simulink model "matlab_ppg_v2"  (R2018a)
settings: Solver=FixedStepAuto  StartTime=0.0  StopTime=inf  RelTol=1e-3  EnableMultiTasking=on
libraries: dspstat3 x5, arduinolib x1, dspsrcs4 x1
settings Model: ExtModeTrigDuration=2  Creator=Na-Teng  LastModifiedBy=Na-Teng
settings OptimizationCC: EnhancedBackFolding=on  PassReuseOutputArgsAs=Individual arguments  MaxStackSize=64  OptimizeBlockOrder=speed  DifferentSizesBufferReuse=on  OptimizationCustomize=off
settings DebuggingCC: ParameterTunabilityLossMsg=error
settings HardwareCC: ProdBitPerInt=16  ProdBitPerPointer=16  ProdBitPerSizeT=16  ProdBitPerPtrDiffT=16  ProdLargestAtomicFloat=None  ProdWordSize=8  ProdHWDeviceType=Atmel->AVR
settings SFSimCC: MATLABDynamicMemAlloc=off
settings RTWCC: SystemTargetFile=ert.tlc  HardwareBoard=Arduino Mega 2560  TLCOptions=-aInlineSetEventsForThisBaseRateFcn=TLC_FALSE -aSuppressMultiTaskScheduler=TLC_FALSE -aRateBasedStepFcn=1  TemplateMakefile=ert_default_tmf  GenerateReport=on  Toolchain=Arduino AVR  BuildConfiguration=Faster Runs  IncludeHyperlinkInReport=on  LaunchReport=on  GenerateTraceInfo=on  GenerateTraceReport=on  GenerateTraceReportSl=on  GenerateTraceReportSf=on  GenerateTraceReportEml=on
settings CodeAppCC: ForceParamTrailComments=on  IgnoreCustomStorageClasses=off  OperatorAnnotations=on  SimulinkDataObjDesc=on  SFDataObjDesc=on  InsertBlockDesc=on
settings ERTTargetCC: SupportContinuousTime=on  SupportVariableSizeSignals=on

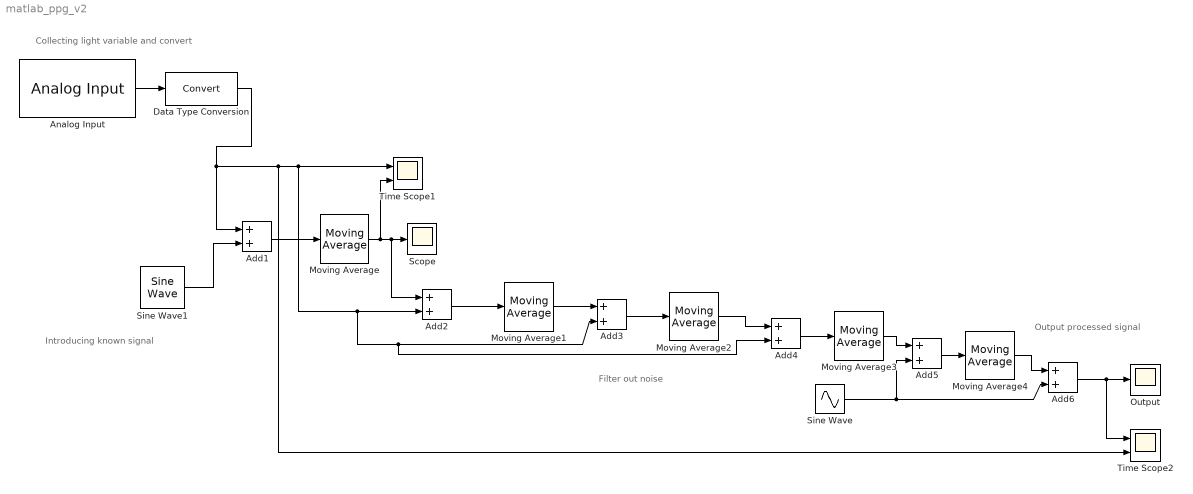
== system matlab_ppg_v2 ==
  note: Output processed signal
  note: Filter out noise
  note: Introducing known signal
  note: Collecting light variable and convert
  Add{1..6} (6 alike) : Sum
  Analog Input : arduinolib/Analog Input  pinNumber=4  ReadResultsOnly=off  ConversionTriggerSource=Software  ExternalTriggerType=uint32(0)  OutputDataType=uint16  EnableConversionCompleteNotify=off  EnableOuputStatus=off  SampleTime=0.001  blockPlatform=arduino
  Data Type Conversion : DataTypeConversion
  Moving Average{,1..4} (5 alike) : dspstat3/Moving Average  Method=Exponential weighting  ForgettingFactorPort=off  SpecifyWindowLength=on  WindowLength=12  ForgettingFactor=0.9  SimulateUsing=Code generation
  "Output " : Scope
  Scope : Scope
  Sine Wave : Sin  SampleTime=0
  Sine Wave1 : dspsrcs4/Sine Wave  Amplitude=1  Frequency=100  Phase=0  SampleMode=Continuous  OutComplex=Real  CompMethod=Trigonometric fcn  TableSize=Speed  SampleTime=0.001  SamplesPerFrame=1  ResetState=Restart at time zero  OutputFrames=off  dataType=double  wordLen=16  udDataType=sfix(16)  fracBitsMode=Best precision  numFracBits=15  OutDataTypeStr=double  LastOutDataTypeStr=double
  Time Scope1 : Scope  NumInputPorts=2
  Time Scope2 : Scope  NumInputPorts=2
  wires:
  Analog Input/1 -> Data Type Conversion/1
  Data Type Conversion/1 -> Add1/1, Time Scope2/2, Time Scope1/1, Add4/2, Add3/2, Add2/2
  Add1/1 -> Moving Average/1
  Moving Average/1 -> Scope/1, Add2/1, Time Scope1/2
  Add2/1 -> Moving Average1/1
  Moving Average1/1 -> Add3/1
  Add3/1 -> Moving Average2/1
  Moving Average2/1 -> Add4/1
  Sine Wave1/1 -> Add1/2
  Add4/1 -> Moving Average3/1
  Moving Average3/1 -> Add5/1
  Sine Wave/1 -> Add6/2, Add5/2
  Add5/1 -> Moving Average4/1
  Moving Average4/1 -> Add6/1
  Add6/1 -> Time Scope2/1, "Output "/1
